simulink model "con_ESTbouncing"  (R2017a)
settings: Solver=FixedStepAuto  StartTime=0.0  StopTime=10.0  FixedStep=0.1  RelTol=1e-3
settings Model: Creator=xiaodong  LastModifiedBy=Sheldon
settings DataIOCC: SaveOutput=off  SignalLogging=off  DSMLogging=off  SaveTime=off

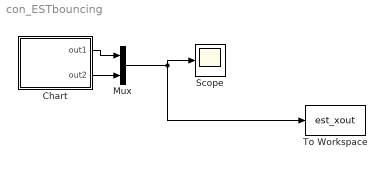
== system con_ESTbouncing ==
  Chart : Stateflow chart  TreatAsAtomicUnit=on
  Mux : Mux  Inputs=2
  Scope : Scope
  To Workspace : ToWorkspace  VariableName=est_xout  SampleTime=0.1
  wires:
  Mux/1 -> Scope/1, To Workspace/1
  Chart/2(out2) -> Mux/2
  Chart/1(out1) -> Mux/1

== stateflow chart con_ESTbouncing/Chart ==
  settings: updateMethod=CONTINUOUS
  state S1
    entry:
    A=[0,1; 0, 0];
    B=[0; -9.810];
    during:
    x1_dot =A(1,1)*x1+A(1,2)*x2+B(1);
    x2_dot =A(2,1)*x1+A(2,2)*x2+B(2);
    out1=x1;
    out2=x2;
  (default) -> S1 : {x1 =10; x2=15;}
  S1 -> S1 : [x1<=0]{x1 = 0;x2 = -0.8*x2+0.7848;}
  data: x1 local size=1; x2 local; out1 output; out2 output; A local size=[2,2]; B local size=[2,1]
  data x1 settings: updateMethod=SF_CONTINUOUS_TIME_DATA
  data x2 settings: updateMethod=SF_CONTINUOUS_TIME_DATA
